simulink model "Adaptive_Control_KpKd"  (R2021b)
settings: Solver=VariableStepAuto  StartTime=0.0  StopTime=10  RelTol=1e-3
undefined symbols (not defined in the file or in its folder): coef_init, Kd, Kp, Kpi, Lambda, q_dq_init
(part 3 of 4)

== matlab function Adaptive_Control_KpKd/Subsystem/Robot ==
  data: q_dq input; dq_ddq output; u input; q output; dq output; g input
function [dq_ddq,q,dq] = fcn(q_dq,u,g)
    q = q_dq(1:length(q_dq)/2);
    dq = q_dq(length(q_dq)/2+1:length(q_dq));
    g_num = g;

%     in1 = q;
%     in2 = [q;dq];
%     in3 = [q;g_num];
%     in1 = mat2cell(in1,ones(numel(in1),1),1);
%     in2 = mat2cell(in2,ones(numel(in2),1),1);
%     in3 = mat2cell(in3,ones(numel(in3),1),1);


    M = M_fun(q);
    C = C_fun(q,dq);
    G = G_fun(q,g_num);

    ddq = M\(u - C - G);
    
    dq_ddq = [dq;ddq];

end
